simulink model "Simulator_tiltrotor"  (R2016b)
settings: Solver=ode45  StartTime=0.0  StopTime=simulation_time  RelTol=1e-3  EnableMultiTasking=on
InitFcn:
  | Parameters_physical_tiltrotor
undefined symbols (not defined in the file or in its folder): A_Servo, B_Servo, C_Servo, delay_attitude, delay_position, dLMN, gravity, inertia_rotor_hub, inertia_tensor, inertia_tensor_inv, Kq, Kt, mass, mass_matrix, mass_matrix_inv, motor_ome_vs_throttle, motor_tau, sample_time, sigbuilder_block
libraries: aerolibutil x10
(part 1 of 2)
settings Model: Creator=Mattia  LastModifiedBy=Mattia
settings DataIOCC: SaveFormat=Array
settings OptimizationCC: LifeSpan=inf
settings DebuggingCC: SFUnexpectedBacktrackingDiag=warning  SFNoUnconditionalDefaultTransitionDiag=warning  SFExecutionAtInitializationDiag=none
settings GRTTargetCC: TargetLangStandard=C89/C90 (ANSI)  GeneratePreprocessorConditionals=Disable all
settings ConfigComp: CovMetricSettings=dw  CovHtmlReporting=on  CovSaveCumulativeToWorkspaceVar=on  CovSaveSingleToWorkspaceVar=on  CovExternalEMLEnable=off

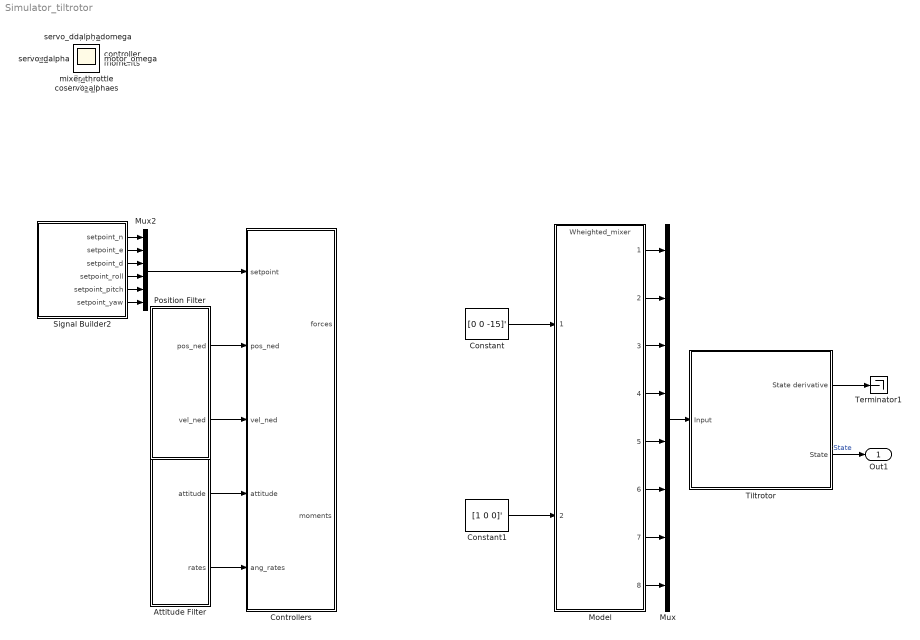
== system Simulator_tiltrotor ==
  Attitude Filter : Subsystem
  Constant : Constant  Value=[0 0 -15]'
  Constant1 : Constant  Value=[1 0 0]'
  Controllers : Subsystem
  Model : ModelReference  ModelNameDialog=Wheighted_mixer.slx  SimulationMode=Normal  ModelReferenceVersion=1.41
  Mux : Mux  Inputs=8
  Mux2 : Mux  Inputs=6
  Position Filter : Subsystem
  Signal Builder2 : Subsystem  Tag=STV Subsys  LoadFcn=sigbuilder_block('load');  StartFcn=sigbuilder_block('start');  StopFcn=sigbuilder_block('stop');  ClipboardFcn=sigbuilder_block('clipboard');  mask(Sigbuilder block){tuvar=[0:10]}
      mask help: Simulink:masks:SigbuilderBlock_MD
      mask init:
      | if ~strcmp(get_param(bdroot(gcbh),'SimulationStatus'),'stopped') tuvar = sigbuilder_block('maskInit'); end
      settings: CopyFcn=sigbuilder_block('copy');  DeleteFcn=sigbuilder_block('delete');  ModelCloseFcn=sigbuilder_block('modelClose');  PreSaveFcn=sigbuilder_block('preSave');  PauseFcn=sigbuilder_block('pause');  ContinueFcn=sigbuilder_block('continue');  NameChangeFcn=sigbuilder_block('namechange');  OpenFcn=sigbuilder_block('open',[6 30 1012.5 447.75 ]);  CloseFcn=sigbuilder_block('close');
      mask Display: plot(0, 0, 100, 100,[2, 2, 32, 32, 2], [68, 8, 8, 68, 68],[32, 2], [38, 38], [32, 19, 2],[53, 60, 44], [32, 17, 17, 2],[16, 16, 31, 31]);txt = getActiveGroup(gcbh);text(2, 100, txt,'verticalAlignment', 'top');
  Terminator1 : Terminator
  Tiltrotor : Subsystem
      mask Display:
      | image(imread('tilt.png'))
      | port_label('input',1,'u')
      | port_label('output',1,'Xdot')
      | port_label('output',2,'X')
  Out1 : Outport
  Fprops : Scope
  Mprops : Scope
  controller_forces : Scope
  controller_moments : Scope
  mixer_alpha : Scope
  mixer_throttle : Scope
  motor_domega : Scope
  motor_omega : Scope
  servo_alpha : Scope
  servo_dalpha : Scope
  servo_ddalpha : Scope
  wires:
  Tiltrotor/1(State derivative) -> Terminator1/1
  Mux/1 -> Tiltrotor/1(Input)
  Tiltrotor/2(State) -> Out1/1  "State"
  Model/1 -> Mux/1
  Model/2 -> Mux/2
  Model/3 -> Mux/3
  Model/4 -> Mux/4
  Model/5 -> Mux/5
  Model/6 -> Mux/6
  Model/7 -> Mux/7
  Model/8 -> Mux/8
  Mux2/1 -> Controllers/1(setpoint)
  Attitude Filter/1(attitude) -> Controllers/4(attitude)
  Attitude Filter/2(rates) -> Controllers/5(ang_rates)
  Position Filter/1(pos_ned) -> Controllers/2(pos_ned)
  Position Filter/2(vel_ned) -> Controllers/3(vel_ned)
  Signal Builder2/3(setpoint_d) -> Mux2/3
  Signal Builder2/4("setpoint_roll ") -> Mux2/4
  Signal Builder2/5(setpoint_pitch) -> Mux2/5
  Signal Builder2/6(setpoint_yaw) -> Mux2/6
  Signal Builder2/2(setpoint_e) -> Mux2/2
  Signal Builder2/1(setpoint_n) -> Mux2/1
  Constant1/1 -> Model/2
  Constant/1 -> Model/1

== system Simulator_tiltrotor/Attitude Filter ==
  Transport Delay : TransportDelay  DelayTime=delay_attitude * sample_time
  Transport Delay1 : TransportDelay  DelayTime=delay_attitude * sample_time
  Zero-Order Hold : ZeroOrderHold  SampleTime=sample_time
  Zero-Order Hold1 : ZeroOrderHold  SampleTime=sample_time
  attitude : Outport  PortDimensions=3
  rates : Outport  Port=2  PortDimensions=3
  wires:
  [ang_rates_body] -> Zero-Order Hold1/1
  [attitude] -> Zero-Order Hold/1
  Zero-Order Hold1/1 -> Transport Delay1/1
  Zero-Order Hold/1 -> Transport Delay/1
  Transport Delay1/1 -> rates/1
  Transport Delay/1 -> attitude/1

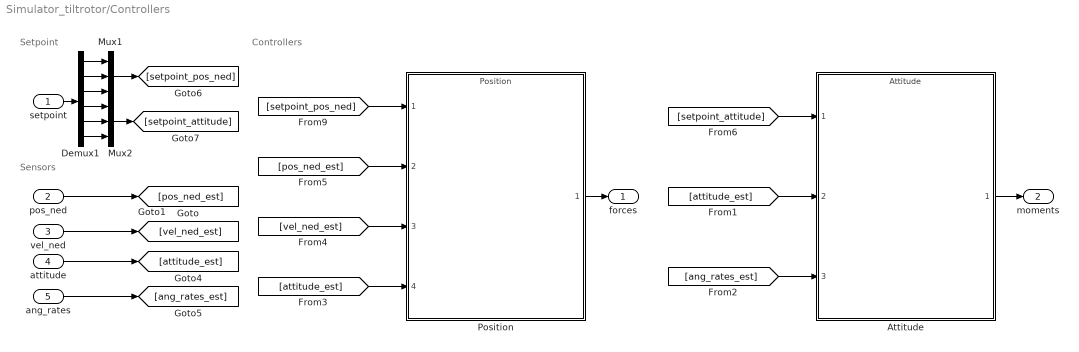
== system Simulator_tiltrotor/Controllers ==
  note: Sensors
  note: Setpoint
  note: Controllers
  setpoint : Inport  PortDimensions=6
  pos_ned : Inport  Port=2  PortDimensions=3
  vel_ned : Inport  Port=3  PortDimensions=3
  attitude : Inport  Port=4  PortDimensions=3
  ang_rates : Inport  Port=5  PortDimensions=3
  Attitude : ModelReference  ModelNameDialog=Attitude.slx  SimulationMode=Normal  ModelReferenceVersion=1.169
  Demux1 : Demux  Outputs=6
  Mux1 : Mux  Inputs=3
  Mux2 : Mux  Inputs=3
  Position : ModelReference  ModelNameDialog=Position.slx  SimulationMode=Normal  ModelReferenceVersion=1.302
  forces : Outport
  moments : Outport  Port=2  PortDimensions=3
  wires:
  setpoint/1 -> Demux1/1
  Demux1/2 -> Mux1/2
  Demux1/1 -> Mux1/1
  [pos_ned_est] -> Position/2
  attitude/1 -> [attitude_est]
  Mux1/1 -> [setpoint_pos_ned]
  [setpoint_pos_ned] -> Position/1
  pos_ned/1 -> [pos_ned_est]
  vel_ned/1 -> [vel_ned_est]
  ang_rates/1 -> [ang_rates_est]
  [attitude_est] -> Position/4
  [vel_ned_est] -> Position/3
  Demux1/3 -> Mux1/3
  Demux1/4 -> Mux2/1
  Demux1/5 -> Mux2/2
  Demux1/6 -> Mux2/3
  Mux2/1 -> [setpoint_attitude]
  Position/1 -> forces/1
  [attitude_est] -> Attitude/2
  Attitude/1 -> moments/1
  [ang_rates_est] -> Attitude/3
  [setpoint_attitude] -> Attitude/1

== system Simulator_tiltrotor/Position Filter ==
  Mux1 : Mux  Inputs=3
  Mux3 : Mux  Inputs=3
  Position NED : Subsystem
  Transport Delay : TransportDelay  DelayTime=delay_position * sample_time
  Transport Delay1 : TransportDelay  DelayTime=delay_position * sample_time
  Velocity NED : Subsystem
  Zero-Order Hold : ZeroOrderHold  SampleTime=sample_time
  Zero-Order Hold1 : ZeroOrderHold  SampleTime=sample_time
  pos_ned : Outport  PortDimensions=3
  vel_ned : Outport  Port=2  PortDimensions=3
  wires:
  Position NED/2(e) -> Mux1/2
  Velocity NED/2(e_vel) -> Mux3/2
  Velocity NED/1(n_vel) -> Mux3/1
  Position NED/1(n) -> Mux1/1
  Zero-Order Hold/1 -> Transport Delay/1
  Mux1/1 -> Zero-Order Hold/1
  Transport Delay/1 -> pos_ned/1
  Zero-Order Hold1/1 -> Transport Delay1/1
  Mux3/1 -> Zero-Order Hold1/1
  Transport Delay1/1 -> vel_ned/1
  Position NED/3(d) -> Mux1/3
  Velocity NED/3(d_vel) -> Mux3/3

== system Simulator_tiltrotor/Signal Builder2 ==
  Demux : Demux  Tag=STV Demux  Outputs=6
  FromWs : FromWorkspace  Tag=STV FromWs  VariableName=tuvar  SampleTime=0
      SigBuilderData=|
      | common.afterFinalStr = 'Extrapolate'
      | common.sampleTime = 0
      | dataSet(1).timeRange = [0 50]
      | dataSet(1).name = 'setpoint'
      | dataSet(2).timeRange = [0 50]
      | dataSet(2).name = 'setpoint_2'
      | sbobj.Groups(1).Name = 'setpoint'
      | sbobj.Groups(1).Signals(1).Name = 'setpoint_n'
      | sbobj.Groups(1).Signals(1).XData = [0 10 13 30 33 50]
      | sbobj.Groups(1).Signals(1).YData = [0 0 1 1 0 0]
      | sbobj.Groups(1).Signals(2).Name = 'setpoint_e'
      | sbobj.Groups(1).Signals(2).XData = [0 50]
      | sbobj.Groups(1).Signals(2).YData = [0 0]
      | sbobj.Groups(1).Signals(3).Name = 'setpoint_d'
      | sbobj.Groups(1).Signals(3).XData = [0 50]
      | sbobj.Groups(1).Signals(3).YData = [-1 -1]
      | sbobj.Groups(1).Signals(4).Name = 'setpoint_roll '
      | sbobj.Groups(1).Signals(4).XData = [0 10 40 50]
      | sbobj.Groups(1).Signals(4).YData = [0 0 0 0]
      | sbobj.Groups(1).Signals(5).Name = 'setpoint_pitch'
      | sbobj.Groups(1).Signals(5).XData = [0 15 16 29 30 50]
      | sbobj.Groups(1).Signals(5).YData = [0 0 1 1 0 0]
      | sbobj.Groups(1).Signals(6).Name = 'setpoint_yaw'
      | sbobj.Groups(1).Signals(6).XData = [0 50]
      | sbobj.Groups(1).Signals(6).YData = [0 0]
      | sbobj.Groups(1).TimeRange = [0 50]
      | sbobj.Groups(2).Name = 'setpoint_2'
      | sbobj.Groups(2).Signals(1).Name = 'setpoint_n'
      | sbobj.Groups(2).Signals(1).XData = [0 10 45 45.05 50]
      | sbobj.Groups(2).Signals(1).YData = [0 0 0 0 0]
      | sbobj.Groups(2).Signals(2).Name = 'setpoint_e'
      | sbobj.Groups(2).Signals(2).XData = [0 10 50]
      | sbobj.Groups(2).Signals(2).YData = [0 0 0]
      | sbobj.Groups(2).Signals(3).Name = 'setpoint_d'
      | sbobj.Groups(2).Signals(3).XData = [0 50]
      | sbobj.Groups(2).Signals(3).YData = [-2 -2]
      | sbobj.Groups(2).Signals(4).Name = 'setpoint_roll '
      | sbobj.Groups(2).Signals(4).XData = [0 10 40 50]
      | sbobj.Groups(2).Signals(4).YData = [0 0 0 0]
      | sbobj.Groups(2).Signals(5).Name = 'setpoint_pitch'
      | sbobj.Groups(2).Signals(5).XData = [0 5 6 14 15 50]
      | sbobj.Groups(2).Signals(5).YData = [0 0 0.314159265359 0.314159265359 0 0]
      | sbobj.Groups(2).Signals(6).Name = 'setpoint_yaw'
      | sbobj.Groups(2).Signals(6).XData = [0 50]
      | sbobj.Groups(2).Signals(6).YData = [0 0]
      | sbobj.Groups(2).TimeRange = [0 50]
  setpoint_n : Outport  Tag=STV Outport
  setpoint_e : Outport  Tag=STV Outport  Port=2
  setpoint_d : Outport  Tag=STV Outport  Port=3
  "setpoint_roll " : Outport  Tag=STV Outport  Port=4
  setpoint_pitch : Outport  Tag=STV Outport  Port=5
  setpoint_yaw : Outport  Tag=STV Outport  Port=6
  wires:
  FromWs/1 -> Demux/1
  Demux/1 -> setpoint_n/1
  Demux/2 -> setpoint_e/1
  Demux/3 -> setpoint_d/1
  Demux/4 -> "setpoint_roll "/1
  Demux/5 -> setpoint_pitch/1
  Demux/6 -> setpoint_yaw/1

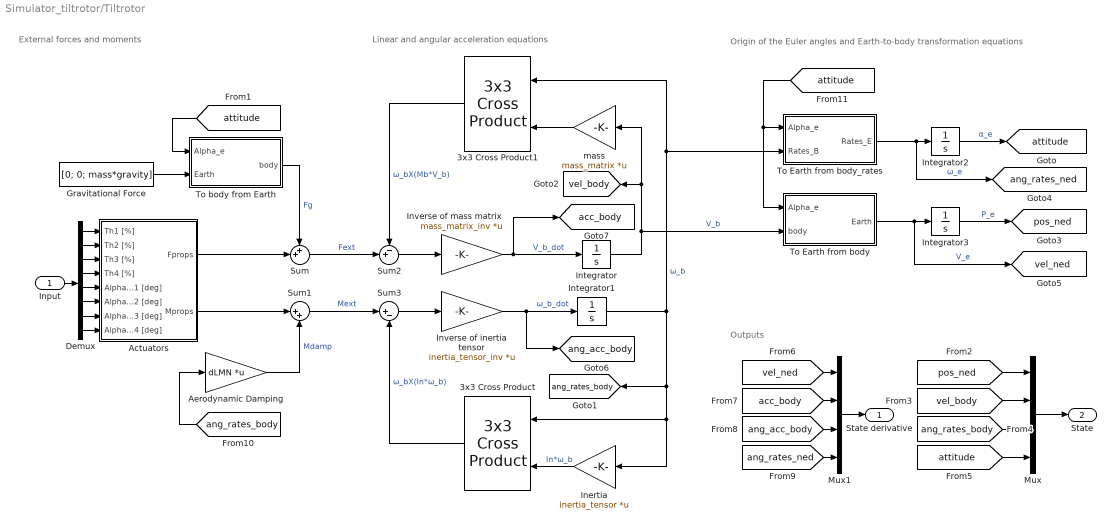
== system Simulator_tiltrotor/Tiltrotor ==
  note: Outputs
  note: Origin of the Euler angles and Earth-to-body transformation equations
  note: Linear and angular acceleration equations
  note: External forces and moments
  Input : Inport
  3x3 Cross Product : aerolibutil/3x3 Cross Product
  3x3 Cross Product1 : aerolibutil/3x3 Cross Product
  Actuators : Subsystem
  Aerodynamic Damping : Gain  Gain=dLMN  Multiplication=Matrix(K*u)
  Demux : Demux  Outputs=8
  Gravitational Force : Constant  Value=[0; 0; mass*gravity]
  Inertia : Gain  Gain=inertia_tensor  Multiplication=Matrix(K*u)
  Integrator{,1..3} (4 alike) : Integrator  InitialCondition=[0; 0; 0]
  Inverse of inertia tensor : Gain  Gain=inertia_tensor_inv  Multiplication=Matrix(K*u)
  Inverse of mass matrix : Gain  Gain=mass_matrix_inv  Multiplication=Matrix(K*u)
  Mux : Mux
  Mux1 : Mux
  Sum : Sum  Inputs=++|
  Sum1 : Sum  Inputs=|++
  Sum2 : Sum  Inputs=-+|
  Sum3 : Sum  Inputs=|+-
  To Earth from body : MATLAB Function  TreatAsAtomicUnit=on
  To Earth from body_rates : MATLAB Function  TreatAsAtomicUnit=on
  To body from Earth : MATLAB Function  TreatAsAtomicUnit=on
  mass : Gain  Gain=mass_matrix  Multiplication=Matrix(K*u)
  State derivative : Outport
  State : Outport  Port=2
  tag scope: acc_body=global, ang_acc_body=global, ang_rates_body=global, ang_rates_ned=global, attitude=global, pos_ned=global, vel_body=global, vel_ned=global
  wires:
  To Earth from body_rates/1(Rates_E) -> Integrator2/1, [ang_rates_ned]  "ω_e"
  [pos_ned] -> Mux/1
  3x3 Cross Product/1 -> Sum3/2  "ω_bX(In*ω_b)"
  [acc_body] -> Mux1/2
  Mux/1 -> State/1
  Mux1/1 -> State derivative/1
  [vel_body] -> Mux/2
  [attitude] -> Mux/4
  [ang_rates_body] -> Mux/3
  [ang_rates_ned] -> Mux1/4
  [ang_acc_body] -> Mux1/3
  [vel_ned] -> Mux1/1
  Inverse of mass matrix/1 -> Integrator/1, [acc_body]  "V_b_dot"
  Integrator/1 -> To Earth from body/2(body), mass/1, [vel_body]  "V_b"
  [attitude] -> To Earth from body/1(Alpha_e), To Earth from body_rates/1(Alpha_e)
  Integrator1/1 -> To Earth from body_rates/2(Rates_B), 3x3 Cross Product1/1, 3x3 Cross Product/1, Inertia/1, [ang_rates_body]  "ω_b"
  Sum3/1 -> Inverse of inertia tensor/1
  Sum2/1 -> Inverse of mass matrix/1
  mass/1 -> 3x3 Cross Product1/2
  Sum/1 -> Sum2/2  "Fext"
  Sum1/1 -> Sum3/1  "Mext"
  Inverse of inertia tensor/1 -> Integrator1/1, [ang_acc_body]  "ω_b_dot"
  3x3 Cross Product1/1 -> Sum2/1  "ω_bX(Mb*V_b)"
  Integrator2/1 -> [attitude]  "α_e"
  Aerodynamic Damping/1 -> Sum1/2  "Mdamp"
  Integrator3/1 -> [pos_ned]  "P_e"
  Inertia/1 -> 3x3 Cross Product/2  "In*ω_b"
  [ang_rates_body] -> Aerodynamic Damping/1
  To Earth from body/1(Earth) -> [vel_ned], Integrator3/1  "V_e"
  To body from Earth/1(body) -> Sum/1  "Fg"
  Gravitational Force/1 -> To body from Earth/2(Earth)
  [attitude] -> To body from Earth/1(Alpha_e)
  Demux/4 -> Actuators/4(Th4 [%])
  Demux/3 -> Actuators/3(Th3 [%])
  Demux/1 -> Actuators/1(Th1 [%])
  Demux/2 -> Actuators/2(Th2 [%])
  Input/1 -> Demux/1
  Demux/5 -> Actuators/5(Alpha_1 [deg])
  Demux/6 -> Actuators/6(Alpha_2 [deg])
  Demux/7 -> Actuators/7(Alpha_3 [deg])
  Demux/8 -> Actuators/8(Alpha_4 [deg])
  Actuators/1(Fprops) -> Sum/2
  Actuators/2(Mprops) -> Sum1/1

== system Simulator_tiltrotor/Position Filter/Position NED ==
  Demux : Demux  Outputs=3
  n : Outport
  e : Outport  Port=2
  d : Outport  Port=3
  wires:
  Demux/1 -> n/1  "n"
  Demux/3 -> d/1  "d"
  [pos_ned] -> Demux/1
  Demux/2 -> e/1  "e"

== system Simulator_tiltrotor/Position Filter/Velocity NED ==
  Demux : Demux  Outputs=3
  n_vel : Outport
  e_vel : Outport  Port=2
  d_vel : Outport  Port=3
  wires:
  Demux/2 -> e_vel/1  "e"
  [vel_ned] -> Demux/1
  Demux/3 -> d_vel/1  "d"
  Demux/1 -> n_vel/1  "n"

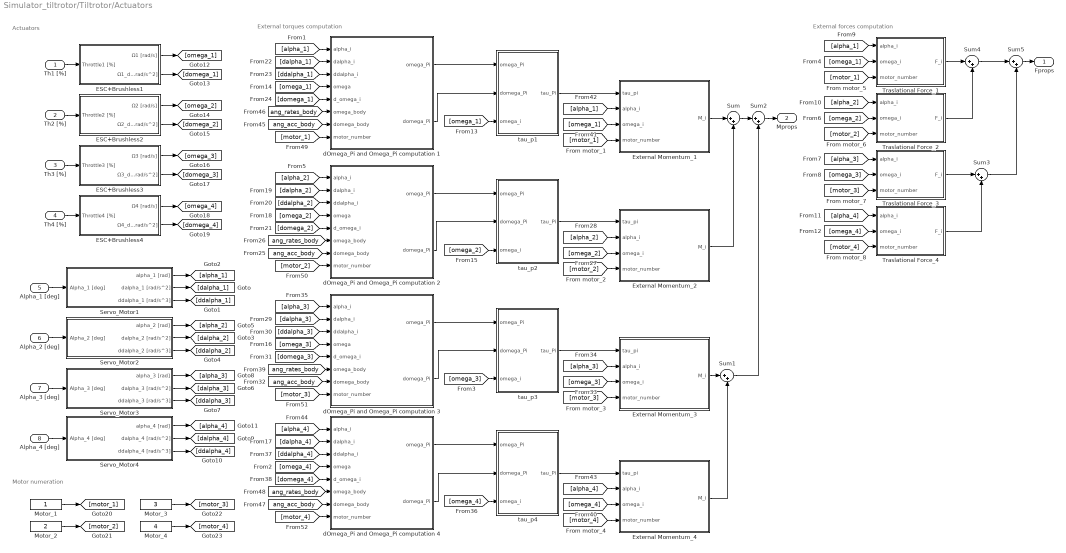
== system Simulator_tiltrotor/Tiltrotor/Actuators ==
  note: Actuators
  note: Motor numeration
  note: External torques computation
  note: External forces computation
  Th1 [%] : Inport
  Th2 [%] : Inport  Port=2
  Th3 [%] : Inport  Port=3
  Th4 [%] : Inport  Port=4
  Alpha_1 [deg] : Inport  Port=5
  Alpha_2 [deg] : Inport  Port=6
  Alpha_3 [deg] : Inport  Port=7
  Alpha_4 [deg] : Inport  Port=8
  ESC+Brushless1 : Subsystem
  ESC+Brushless2 : Subsystem
  ESC+Brushless3 : Subsystem
  ESC+Brushless4 : Subsystem
  External Momentum_1 : Subsystem
  External Momentum_2 : Subsystem
  External Momentum_3 : Subsystem
  External Momentum_4 : Subsystem
  Motor_1 : Constant
  Motor_2 : Constant  Value=2
  Motor_3 : Constant  Value=3
  Motor_4 : Constant  Value=4
  Servo_Motor1 : Subsystem
  Servo_Motor2 : Subsystem
  Servo_Motor3 : Subsystem
  Servo_Motor4 : Subsystem
  Sum{,1..5} (6 alike) : Sum  Inputs=|++
  Traslational Force_1 : Subsystem
  Traslational Force_2 : Subsystem
  Traslational Force_3 : Subsystem
  Traslational Force_4 : Subsystem
  dOmega_Pi and Omega_Pi computation 1 : Subsystem
  dOmega_Pi and Omega_Pi computation 2 : Subsystem
  dOmega_Pi and Omega_Pi computation 3 : Subsystem
  dOmega_Pi and Omega_Pi computation 4 : Subsystem
  tau_p1 : Subsystem
  tau_p2 : Subsystem
  tau_p3 : Subsystem
  tau_p4 : Subsystem
  Fprops : Outport
  Mprops : Outport  Port=2
  wires:
  Th1 [%]/1 -> ESC+Brushless1/1(Throttle1 [%])
  Th2 [%]/1 -> ESC+Brushless2/1(Throttle2 [%])
  Th4 [%]/1 -> ESC+Brushless4/1(Throttle4 [%])
  Th3 [%]/1 -> ESC+Brushless3/1(Throttle3 [%])
  Alpha_1 [deg]/1 -> Servo_Motor1/1(Alpha_1 [deg])
  Servo_Motor1/2(dalpha_1 [rad/s^2]) -> [dalpha_1]
  Servo_Motor1/3(ddalpha_1 [rad/s^3]) -> [ddalpha_1]
  Servo_Motor3/1(alpha_3 [rad]) -> [alpha_3]
  Servo_Motor3/3(ddalpha_3 [rad/s^3]) -> [ddalpha_3]
  Servo_Motor3/2(dalpha_3 [rad/s^2]) -> [dalpha_3]
  Servo_Motor2/3(ddalpha_2 [rad/s^3]) -> [ddalpha_2]
  Servo_Motor2/2(dalpha_2 [rad/s^2]) -> [dalpha_2]
  Servo_Motor2/1(alpha_2 [rad]) -> [alpha_2]
  Servo_Motor1/1(alpha_1 [rad]) -> [alpha_1]
  Servo_Motor4/1(alpha_4 [rad]) -> [alpha_4]
  Servo_Motor4/2(dalpha_4 [rad/s^2]) -> [dalpha_4]
  Servo_Motor4/3(ddalpha_4 [rad/s^3]) -> [ddalpha_4]
  ESC+Brushless1/1(Ω1 [rad/s]) -> [omega_1]
  ESC+Brushless1/2(Ω1_dot [rad/s^2]) -> [domega_1]
  ESC+Brushless2/1(Ω2 [rad/s]) -> [omega_2]
  ESC+Brushless3/1(Ω3 [rad/s]) -> [omega_3]
  ESC+Brushless3/2(Ω3_dot [rad/s^2]) -> [domega_3]
  ESC+Brushless4/1(Ω4 [rad/s]) -> [omega_4]
  ESC+Brushless4/2(Ω4_dot [rad/s^2]) -> [domega_4]
  [alpha_1] -> dOmega_Pi and Omega_Pi computation 1/1(alpha_i)
  [dalpha_1] -> dOmega_Pi and Omega_Pi computation 1/2(dalpha_i)
  [ddalpha_1] -> dOmega_Pi and Omega_Pi computation 1/3(ddalpha_i)
  dOmega_Pi and Omega_Pi computation 1/1(omega_Pi) -> tau_p1/1(omega_Pi)
  dOmega_Pi and Omega_Pi computation 1/2(domega_Pi) -> tau_p1/2(domega_Pi)
  tau_p1/1(tau_Pi) -> External Momentum_1/1(tau_pi)
  [alpha_1] -> External Momentum_1/2(alpha_i)
  [omega_1] -> External Momentum_1/3(omega_i)
  External Momentum_1/1(M_i) -> Sum/1
  Sum/1 -> Sum2/1
  Sum2/1 -> Mprops/1
  [alpha_1] -> Traslational Force_1/1(alpha_i)
  [omega_1] -> Traslational Force_1/2(omega_i)
  Motor_1/1 -> [motor_1]
  Motor_2/1 -> [motor_2]
  Motor_3/1 -> [motor_3]
  Motor_4/1 -> [motor_4]
  Traslational Force_3/1(F_i) -> Sum3/1
  Traslational Force_4/1(F_i) -> Sum3/2
  Traslational Force_1/1(F_i) -> Sum4/1
  Traslational Force_2/1(F_i) -> Sum4/2
  Sum4/1 -> Sum5/1
  Sum3/1 -> Sum5/2
  Sum5/1 -> Fprops/1
  [omega_1] -> tau_p1/3(omega_i)
  Sum1/1 -> Sum2/2
  ESC+Brushless2/2(Ω2_dot [rad/s^2]) -> [domega_2]
  Alpha_2 [deg]/1 -> Servo_Motor2/1(Alpha_2 [deg])
  Alpha_3 [deg]/1 -> Servo_Motor3/1(Alpha_3 [deg])
  Alpha_4 [deg]/1 -> Servo_Motor4/1(Alpha_4 [deg])
  [motor_1] -> External Momentum_1/4(motor_number)
  [alpha_2] -> dOmega_Pi and Omega_Pi computation 2/1(alpha_i)
  [dalpha_2] -> dOmega_Pi and Omega_Pi computation 2/2(dalpha_i)
  [ddalpha_2] -> dOmega_Pi and Omega_Pi computation 2/3(ddalpha_i)
  tau_p2/1(tau_Pi) -> External Momentum_2/1(tau_pi)
  [alpha_2] -> External Momentum_2/2(alpha_i)
  [omega_2] -> External Momentum_2/3(omega_i)
  External Momentum_2/1(M_i) -> Sum/2
  [omega_2] -> tau_p2/3(omega_i)
  [motor_2] -> External Momentum_2/4(motor_number)
  [alpha_3] -> dOmega_Pi and Omega_Pi computation 3/1(alpha_i)
  [dalpha_3] -> dOmega_Pi and Omega_Pi computation 3/2(dalpha_i)
  [ddalpha_3] -> dOmega_Pi and Omega_Pi computation 3/3(ddalpha_i)
  dOmega_Pi and Omega_Pi computation 3/1(omega_Pi) -> tau_p3/1(omega_Pi)
  dOmega_Pi and Omega_Pi computation 3/2(domega_Pi) -> tau_p3/2(domega_Pi)
  [alpha_3] -> External Momentum_3/2(alpha_i)
  [omega_3] -> External Momentum_3/3(omega_i)
  [omega_3] -> tau_p3/3(omega_i)
  [motor_3] -> External Momentum_3/4(motor_number)
  External Momentum_3/1(M_i) -> Sum1/1
  [alpha_4] -> dOmega_Pi and Omega_Pi computation 4/1(alpha_i)
  [dalpha_4] -> dOmega_Pi and Omega_Pi computation 4/2(dalpha_i)
  [ddalpha_4] -> dOmega_Pi and Omega_Pi computation 4/3(ddalpha_i)
  tau_p4/1(tau_Pi) -> External Momentum_4/1(tau_pi)
  [alpha_4] -> External Momentum_4/2(alpha_i)
  [omega_4] -> External Momentum_4/3(omega_i)
  [omega_4] -> tau_p4/3(omega_i)
  [motor_4] -> External Momentum_4/4(motor_number)
  External Momentum_4/1(M_i) -> Sum1/2
  dOmega_Pi and Omega_Pi computation 2/1(omega_Pi) -> tau_p2/1(omega_Pi)
  dOmega_Pi and Omega_Pi computation 2/2(domega_Pi) -> tau_p2/2(domega_Pi)
  [domega_4] -> dOmega_Pi and Omega_Pi computation 4/5(d_omega_i)
  [omega_4] -> dOmega_Pi and Omega_Pi computation 4/4(omega)
  [domega_1] -> dOmega_Pi and Omega_Pi computation 1/5(d_omega_i)
  [omega_1] -> dOmega_Pi and Omega_Pi computation 1/4(omega)
  [ang_rates_body] -> dOmega_Pi and Omega_Pi computation 1/6(omega_body)
  [ang_acc_body] -> dOmega_Pi and Omega_Pi computation 1/7(domega_body)
  [omega_2] -> dOmega_Pi and Omega_Pi computation 2/4(omega)
  [domega_2] -> dOmega_Pi and Omega_Pi computation 2/5(d_omega_i)
  [domega_3] -> dOmega_Pi and Omega_Pi computation 3/5(d_omega_i)
  [omega_3] -> dOmega_Pi and Omega_Pi computation 3/4(omega)
  [ang_rates_body] -> dOmega_Pi and Omega_Pi computation 2/6(omega_body)
  [ang_rates_body] -> dOmega_Pi and Omega_Pi computation 3/6(omega_body)
  [ang_rates_body] -> dOmega_Pi and Omega_Pi computation 4/6(omega_body)
  [ang_acc_body] -> dOmega_Pi and Omega_Pi computation 2/7(domega_body)
  [ang_acc_body] -> dOmega_Pi and Omega_Pi computation 3/7(domega_body)
  [ang_acc_body] -> dOmega_Pi and Omega_Pi computation 4/7(domega_body)
  [motor_1] -> Traslational Force_1/3(motor_number)
  [alpha_2] -> Traslational Force_2/1(alpha_i)
  [alpha_3] -> Traslational Force_3/1(alpha_i)
  [alpha_4] -> Traslational Force_4/1(alpha_i)
  [omega_4] -> Traslational Force_4/2(omega_i)
  [omega_3] -> Traslational Force_3/2(omega_i)
  [motor_2] -> Traslational Force_2/3(motor_number)
  [motor_3] -> Traslational Force_3/3(motor_number)
  [motor_4] -> Traslational Force_4/3(motor_number)
  [omega_2] -> Traslational Force_2/2(omega_i)
  [motor_1] -> dOmega_Pi and Omega_Pi computation 1/8(motor_number)
  dOmega_Pi and Omega_Pi computation 4/1(omega_Pi) -> tau_p4/1(omega_Pi)
  tau_p3/1(tau_Pi) -> External Momentum_3/1(tau_pi)
  dOmega_Pi and Omega_Pi computation 4/2(domega_Pi) -> tau_p4/2(domega_Pi)
  [motor_2] -> dOmega_Pi and Omega_Pi computation 2/8(motor_number)
  [motor_3] -> dOmega_Pi and Omega_Pi computation 3/8(motor_number)
  [motor_4] -> dOmega_Pi and Omega_Pi computation 4/8(motor_number)

== system Simulator_tiltrotor/Tiltrotor/Actuators/ESC+Brushless1 ==
  Throttle1 [%] : Inport
  Gain : Gain
  Gain1 : Gain
  Subsystem : Subsystem
  Ω1 [rad/s] : Outport
  Ω1_dot [rad/s^2] : Outport  Port=2
  wires:
  Subsystem/1(omega_i) -> Gain/1
  Subsystem/2(domega_i) -> Gain1/1
  Throttle1 [%]/1 -> Subsystem/1(Throttle [%])
  Gain/1 -> Ω1 [rad/s]/1
  Gain1/1 -> Ω1_dot [rad/s^2]/1

== system Simulator_tiltrotor/Tiltrotor/Actuators/ESC+Brushless2 ==
  Throttle2 [%] : Inport
  Gain : Gain  Gain=-1
  Gain1 : Gain  Gain=-1
  Subsystem : Subsystem
  Ω2 [rad/s] : Outport
  Ω2_dot [rad/s^2] : Outport  Port=2
  wires:
  Subsystem/1(omega_i) -> Gain/1
  Subsystem/2(domega_i) -> Gain1/1
  Throttle2 [%]/1 -> Subsystem/1(Throttle [%])
  Gain/1 -> Ω2 [rad/s]/1
  Gain1/1 -> Ω2_dot [rad/s^2]/1

== system Simulator_tiltrotor/Tiltrotor/Actuators/ESC+Brushless3 ==
  Throttle3 [%] : Inport
  Gain : Gain
  Gain1 : Gain
  Subsystem : Subsystem
  Ω3 [rad/s] : Outport
  Ω3_dot [rad/s^2] : Outport  Port=2
  wires:
  Subsystem/1(omega_i) -> Gain/1
  Subsystem/2(domega_i) -> Gain1/1
  Throttle3 [%]/1 -> Subsystem/1(Throttle [%])
  Gain/1 -> Ω3 [rad/s]/1
  Gain1/1 -> Ω3_dot [rad/s^2]/1

== system Simulator_tiltrotor/Tiltrotor/Actuators/ESC+Brushless4 ==
  Throttle4 [%] : Inport
  Gain : Gain  Gain=-1
  Gain1 : Gain  Gain=-1
  Subsystem : Subsystem
  Ω4 [rad/s] : Outport
  Ω4_dot [rad/s^2] : Outport  Port=2
  wires:
  Subsystem/1(omega_i) -> Gain/1
  Subsystem/2(domega_i) -> Gain1/1
  Throttle4 [%]/1 -> Subsystem/1(Throttle [%])
  Gain/1 -> Ω4 [rad/s]/1
  Gain1/1 -> Ω4_dot [rad/s^2]/1

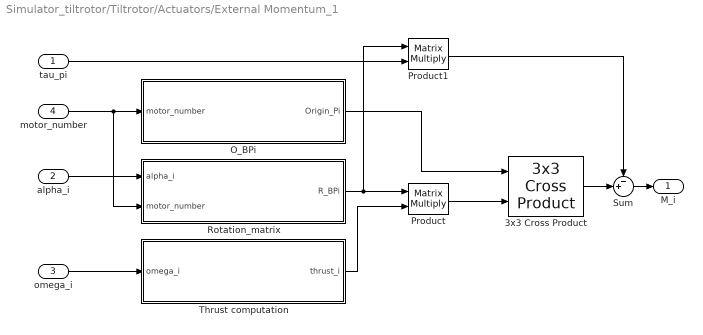
== system Simulator_tiltrotor/Tiltrotor/Actuators/External Momentum_1 ==
  tau_pi : Inport
  alpha_i : Inport  Port=2
  omega_i : Inport  Port=3
  motor_number : Inport  Port=4
  3x3 Cross Product : aerolibutil/3x3 Cross Product
  O_BPi : MATLAB Function  TreatAsAtomicUnit=on
  Product : Product  Multiplication=Matrix(*)
  Product1 : Product  Multiplication=Matrix(*)
  Rotation_matrix : MATLAB Function  TreatAsAtomicUnit=on
  Sum : Sum  Inputs=-+|
  Thrust computation : Subsystem
  M_i : Outport
  wires:
  Sum/1 -> M_i/1
  Rotation_matrix/1(R_BPi) -> Product1/1, Product/1
  alpha_i/1 -> Rotation_matrix/1(alpha_i)
  Product/1 -> 3x3 Cross Product/2
  tau_pi/1 -> Product1/2
  motor_number/1 -> Rotation_matrix/2(motor_number), O_BPi/1(motor_number)
  omega_i/1 -> Thrust computation/1(omega_i)
  Thrust computation/1(thrust_i) -> Product/2
  3x3 Cross Product/1 -> Sum/2
  Product1/1 -> Sum/1
  O_BPi/1(Origin_Pi) -> 3x3 Cross Product/1

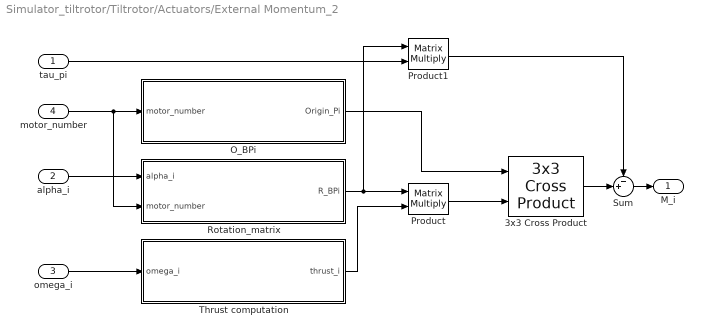
== system Simulator_tiltrotor/Tiltrotor/Actuators/External Momentum_2 ==
  tau_pi : Inport
  alpha_i : Inport  Port=2
  omega_i : Inport  Port=3
  motor_number : Inport  Port=4
  3x3 Cross Product : aerolibutil/3x3 Cross Product
  O_BPi : MATLAB Function  TreatAsAtomicUnit=on
  Product : Product  Multiplication=Matrix(*)
  Product1 : Product  Multiplication=Matrix(*)
  Rotation_matrix : MATLAB Function  TreatAsAtomicUnit=on
  Sum : Sum  Inputs=-+|
  Thrust computation : Subsystem
  M_i : Outport
  wires:
  Sum/1 -> M_i/1
  Rotation_matrix/1(R_BPi) -> Product1/1, Product/1
  alpha_i/1 -> Rotation_matrix/1(alpha_i)
  Product/1 -> 3x3 Cross Product/2
  tau_pi/1 -> Product1/2
  motor_number/1 -> Rotation_matrix/2(motor_number), O_BPi/1(motor_number)
  omega_i/1 -> Thrust computation/1(omega_i)
  Thrust computation/1(thrust_i) -> Product/2
  3x3 Cross Product/1 -> Sum/2
  Product1/1 -> Sum/1
  O_BPi/1(Origin_Pi) -> 3x3 Cross Product/1

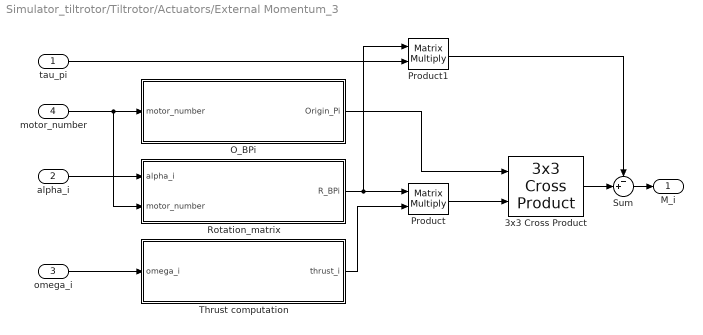
== system Simulator_tiltrotor/Tiltrotor/Actuators/External Momentum_3 ==
  tau_pi : Inport
  alpha_i : Inport  Port=2
  omega_i : Inport  Port=3
  motor_number : Inport  Port=4
  3x3 Cross Product : aerolibutil/3x3 Cross Product
  O_BPi : MATLAB Function  TreatAsAtomicUnit=on
  Product : Product  Multiplication=Matrix(*)
  Product1 : Product  Multiplication=Matrix(*)
  Rotation_matrix : MATLAB Function  TreatAsAtomicUnit=on
  Sum : Sum  Inputs=-+|
  Thrust computation : Subsystem
  M_i : Outport
  wires:
  Sum/1 -> M_i/1
  Rotation_matrix/1(R_BPi) -> Product1/1, Product/1
  alpha_i/1 -> Rotation_matrix/1(alpha_i)
  Product/1 -> 3x3 Cross Product/2
  tau_pi/1 -> Product1/2
  motor_number/1 -> Rotation_matrix/2(motor_number), O_BPi/1(motor_number)
  omega_i/1 -> Thrust computation/1(omega_i)
  Thrust computation/1(thrust_i) -> Product/2
  3x3 Cross Product/1 -> Sum/2
  Product1/1 -> Sum/1
  O_BPi/1(Origin_Pi) -> 3x3 Cross Product/1

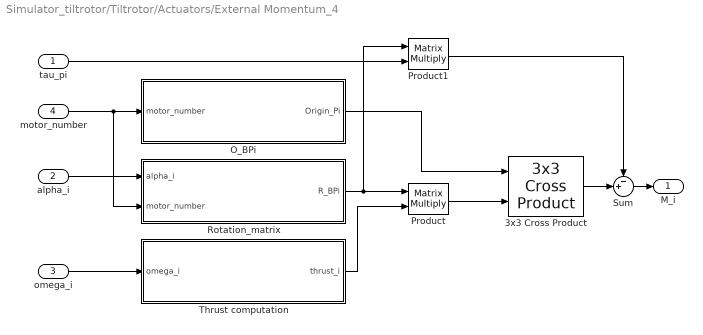
== system Simulator_tiltrotor/Tiltrotor/Actuators/External Momentum_4 ==
  tau_pi : Inport
  alpha_i : Inport  Port=2
  omega_i : Inport  Port=3
  motor_number : Inport  Port=4
  3x3 Cross Product : aerolibutil/3x3 Cross Product
  O_BPi : MATLAB Function  TreatAsAtomicUnit=on
  Product : Product  Multiplication=Matrix(*)
  Product1 : Product  Multiplication=Matrix(*)
  Rotation_matrix : MATLAB Function  TreatAsAtomicUnit=on
  Sum : Sum  Inputs=-+|
  Thrust computation : Subsystem
  M_i : Outport
  wires:
  Sum/1 -> M_i/1
  Rotation_matrix/1(R_BPi) -> Product1/1, Product/1
  alpha_i/1 -> Rotation_matrix/1(alpha_i)
  Product/1 -> 3x3 Cross Product/2
  tau_pi/1 -> Product1/2
  motor_number/1 -> Rotation_matrix/2(motor_number), O_BPi/1(motor_number)
  omega_i/1 -> Thrust computation/1(omega_i)
  Thrust computation/1(thrust_i) -> Product/2
  3x3 Cross Product/1 -> Sum/2
  Product1/1 -> Sum/1
  O_BPi/1(Origin_Pi) -> 3x3 Cross Product/1

== system Simulator_tiltrotor/Tiltrotor/Actuators/Servo_Motor1 ==
  Alpha_1 [deg] : Inport
  Demux : Demux  Outputs=3
  State-Space : StateSpace  A=A_Servo  B=B_Servo  C=C_Servo  D=[0 0 0]'  X0=[0 0 0 ]  ContinuousStateAttributes=['alpha' 'dalpha' 'ddalpha']
  deg2rad : Gain  Gain=deg2rad
  alpha_1 [rad] : Outport
  dalpha_1 [rad/s^2] : Outport  Port=2
  ddalpha_1 [rad/s^3] : Outport  Port=3
  wires:
  deg2rad/1 -> State-Space/1
  Alpha_1 [deg]/1 -> deg2rad/1
  State-Space/1 -> Demux/1
  Demux/1 -> alpha_1 [rad]/1
  Demux/2 -> dalpha_1 [rad/s^2]/1
  Demux/3 -> ddalpha_1 [rad/s^3]/1

== system Simulator_tiltrotor/Tiltrotor/Actuators/Servo_Motor2 ==
  Alpha_2 [deg] : Inport
  Demux : Demux  Outputs=3
  State-Space : StateSpace  A=A_Servo  B=B_Servo  C=C_Servo  D=[0 0 0]'  X0=[0 0 0 ]  ContinuousStateAttributes=['alpha' 'dalpha' 'ddalpha']
  deg2rad : Gain  Gain=deg2rad
  alpha_2 [rad] : Outport
  dalpha_2 [rad/s^2] : Outport  Port=2
  ddalpha_2 [rad/s^3] : Outport  Port=3
  wires:
  deg2rad/1 -> State-Space/1
  Alpha_2 [deg]/1 -> deg2rad/1
  State-Space/1 -> Demux/1
  Demux/1 -> alpha_2 [rad]/1
  Demux/2 -> dalpha_2 [rad/s^2]/1
  Demux/3 -> ddalpha_2 [rad/s^3]/1

== system Simulator_tiltrotor/Tiltrotor/Actuators/Servo_Motor3 ==
  Alpha_3 [deg] : Inport
  Demux : Demux  Outputs=3
  State-Space : StateSpace  A=A_Servo  B=B_Servo  C=C_Servo  D=[0 0 0]'  X0=[0 0 0 ]  ContinuousStateAttributes=['alpha' 'dalpha' 'ddalpha']
  deg2rad : Gain  Gain=deg2rad
  alpha_3 [rad] : Outport
  dalpha_3 [rad/s^2] : Outport  Port=2
  ddalpha_3 [rad/s^3] : Outport  Port=3
  wires:
  deg2rad/1 -> State-Space/1
  Alpha_3 [deg]/1 -> deg2rad/1
  State-Space/1 -> Demux/1
  Demux/1 -> alpha_3 [rad]/1
  Demux/2 -> dalpha_3 [rad/s^2]/1
  Demux/3 -> ddalpha_3 [rad/s^3]/1

== system Simulator_tiltrotor/Tiltrotor/Actuators/Servo_Motor4 ==
  Alpha_4 [deg] : Inport
  Demux : Demux  Outputs=3
  State-Space : StateSpace  A=A_Servo  B=B_Servo  C=C_Servo  D=[0 0 0]'  X0=[0 0 0 ]  ContinuousStateAttributes=['alpha' 'dalpha' 'ddalpha']
  deg2rad : Gain  Gain=deg2rad
  alpha_4 [rad] : Outport
  dalpha_4 [rad/s^2] : Outport  Port=2
  ddalpha_4 [rad/s^3] : Outport  Port=3
  wires:
  deg2rad/1 -> State-Space/1
  Alpha_4 [deg]/1 -> deg2rad/1
  State-Space/1 -> Demux/1
  Demux/1 -> alpha_4 [rad]/1
  Demux/2 -> dalpha_4 [rad/s^2]/1
  Demux/3 -> ddalpha_4 [rad/s^3]/1

== system Simulator_tiltrotor/Tiltrotor/Actuators/Traslational Force_1 ==
  alpha_i : Inport
  omega_i : Inport  Port=2
  motor_number : Inport  Port=3
  Product : Product  Multiplication=Matrix(*)
  Rotation_matrix : MATLAB Function  TreatAsAtomicUnit=on
  Thrust computation : Subsystem
  F_i : Outport
  wires:
  Thrust computation/1(thrust_i) -> Product/2
  Product/1 -> F_i/1
  omega_i/1 -> Thrust computation/1(omega_i)
  Rotation_matrix/1(R_BPi) -> Product/1
  alpha_i/1 -> Rotation_matrix/1(alpha_i)
  motor_number/1 -> Rotation_matrix/2(motor_number)

== system Simulator_tiltrotor/Tiltrotor/Actuators/Traslational Force_2 ==
  alpha_i : Inport
  omega_i : Inport  Port=2
  motor_number : Inport  Port=3
  Product : Product  Multiplication=Matrix(*)
  Rotation_matrix : MATLAB Function  TreatAsAtomicUnit=on
  Thrust computation : Subsystem
  F_i : Outport
  wires:
  motor_number/1 -> Rotation_matrix/2(motor_number)
  alpha_i/1 -> Rotation_matrix/1(alpha_i)
  Rotation_matrix/1(R_BPi) -> Product/1
  omega_i/1 -> Thrust computation/1(omega_i)
  Product/1 -> F_i/1
  Thrust computation/1(thrust_i) -> Product/2

== system Simulator_tiltrotor/Tiltrotor/Actuators/Traslational Force_3 ==
  alpha_i : Inport
  omega_i : Inport  Port=2
  motor_number : Inport  Port=3
  Product : Product  Multiplication=Matrix(*)
  Rotation_matrix : MATLAB Function  TreatAsAtomicUnit=on
  Thrust computation : Subsystem
  F_i : Outport
  wires:
  Thrust computation/1(thrust_i) -> Product/2
  Product/1 -> F_i/1
  omega_i/1 -> Thrust computation/1(omega_i)
  Rotation_matrix/1(R_BPi) -> Product/1
  alpha_i/1 -> Rotation_matrix/1(alpha_i)
  motor_number/1 -> Rotation_matrix/2(motor_number)

== system Simulator_tiltrotor/Tiltrotor/Actuators/Traslational Force_4 ==
  alpha_i : Inport
  omega_i : Inport  Port=2
  motor_number : Inport  Port=3
  Product : Product  Multiplication=Matrix(*)
  Rotation_matrix : MATLAB Function  TreatAsAtomicUnit=on
  Thrust computation : Subsystem
  F_i : Outport
  wires:
  motor_number/1 -> Rotation_matrix/2(motor_number)
  alpha_i/1 -> Rotation_matrix/1(alpha_i)
  Rotation_matrix/1(R_BPi) -> Product/1
  omega_i/1 -> Thrust computation/1(omega_i)
  Product/1 -> F_i/1
  Thrust computation/1(thrust_i) -> Product/2

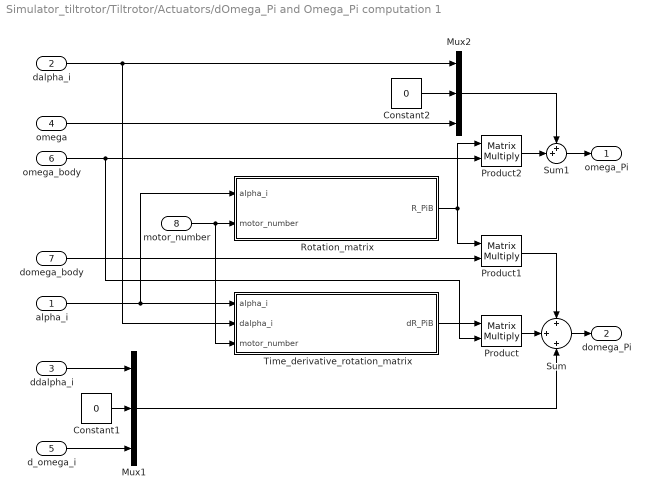
== system Simulator_tiltrotor/Tiltrotor/Actuators/dOmega_Pi and Omega_Pi computation 1 ==
  alpha_i : Inport
  dalpha_i : Inport  Port=2
  ddalpha_i : Inport  Port=3
  omega : Inport  Port=4
  d_omega_i : Inport  Port=5
  omega_body : Inport  Port=6
  domega_body : Inport  Port=7
  motor_number : Inport  Port=8
  Constant1 : Constant  Value=0
  Constant2 : Constant  Value=0
  Mux1 : Mux  Inputs=3
  Mux2 : Mux  Inputs=3
  Product : Product  Multiplication=Matrix(*)
  Product1 : Product  Multiplication=Matrix(*)
  Product2 : Product  Multiplication=Matrix(*)
  Rotation_matrix : MATLAB Function  TreatAsAtomicUnit=on
  Sum : Sum  Inputs=+|+|+
  Sum1 : Sum  Inputs=++|
  Time_derivative_rotation_matrix : MATLAB Function  TreatAsAtomicUnit=on
  omega_Pi : Outport
  domega_Pi : Outport  Port=2
  wires:
  domega_body/1 -> Product1/2
  Product/1 -> Sum/2
  Time_derivative_rotation_matrix/1(dR_PiB) -> Product/1
  Constant1/1 -> Mux1/2
  omega_body/1 -> Product2/2, Product/2
  dalpha_i/1 -> Time_derivative_rotation_matrix/2(dalpha_i), Mux2/1
  alpha_i/1 -> Time_derivative_rotation_matrix/1(alpha_i), Rotation_matrix/1(alpha_i)
  Rotation_matrix/1(R_PiB) -> Product2/1, Product1/1
  Sum/1 -> domega_Pi/1
  Product1/1 -> Sum/1
  Mux1/1 -> Sum/3
  ddalpha_i/1 -> Mux1/1
  Product2/1 -> Sum1/2
  Constant2/1 -> Mux2/2
  Mux2/1 -> Sum1/1
  Sum1/1 -> omega_Pi/1
  d_omega_i/1 -> Mux1/3
  omega/1 -> Mux2/3
  motor_number/1 -> Rotation_matrix/2(motor_number), Time_derivative_rotation_matrix/3(motor_number)

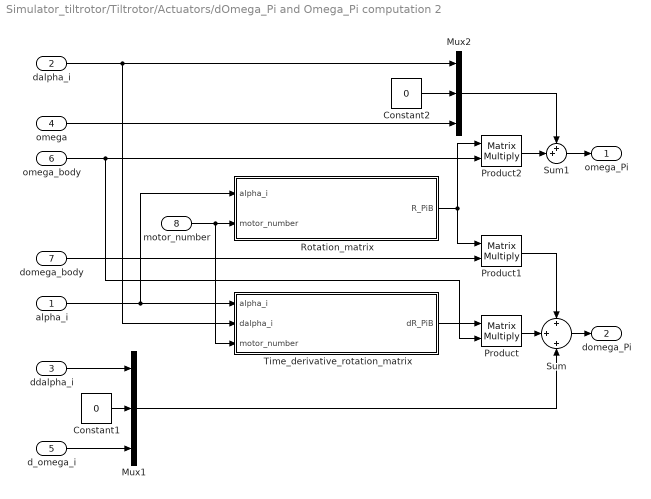
== system Simulator_tiltrotor/Tiltrotor/Actuators/dOmega_Pi and Omega_Pi computation 2 ==
  alpha_i : Inport
  dalpha_i : Inport  Port=2
  ddalpha_i : Inport  Port=3
  omega : Inport  Port=4
  d_omega_i : Inport  Port=5
  omega_body : Inport  Port=6
  domega_body : Inport  Port=7
  motor_number : Inport  Port=8
  Constant1 : Constant  Value=0
  Constant2 : Constant  Value=0
  Mux1 : Mux  Inputs=3
  Mux2 : Mux  Inputs=3
  Product : Product  Multiplication=Matrix(*)
  Product1 : Product  Multiplication=Matrix(*)
  Product2 : Product  Multiplication=Matrix(*)
  Rotation_matrix : MATLAB Function  TreatAsAtomicUnit=on
  Sum : Sum  Inputs=+|+|+
  Sum1 : Sum  Inputs=++|
  Time_derivative_rotation_matrix : MATLAB Function  TreatAsAtomicUnit=on
  omega_Pi : Outport
  domega_Pi : Outport  Port=2
  wires:
  domega_body/1 -> Product1/2
  Product/1 -> Sum/2
  Time_derivative_rotation_matrix/1(dR_PiB) -> Product/1
  Constant1/1 -> Mux1/2
  omega_body/1 -> Product2/2, Product/2
  dalpha_i/1 -> Time_derivative_rotation_matrix/2(dalpha_i), Mux2/1
  alpha_i/1 -> Time_derivative_rotation_matrix/1(alpha_i), Rotation_matrix/1(alpha_i)
  Rotation_matrix/1(R_PiB) -> Product2/1, Product1/1
  Sum/1 -> domega_Pi/1
  Product1/1 -> Sum/1
  Mux1/1 -> Sum/3
  ddalpha_i/1 -> Mux1/1
  Product2/1 -> Sum1/2
  Constant2/1 -> Mux2/2
  Mux2/1 -> Sum1/1
  Sum1/1 -> omega_Pi/1
  d_omega_i/1 -> Mux1/3
  omega/1 -> Mux2/3
  motor_number/1 -> Rotation_matrix/2(motor_number), Time_derivative_rotation_matrix/3(motor_number)

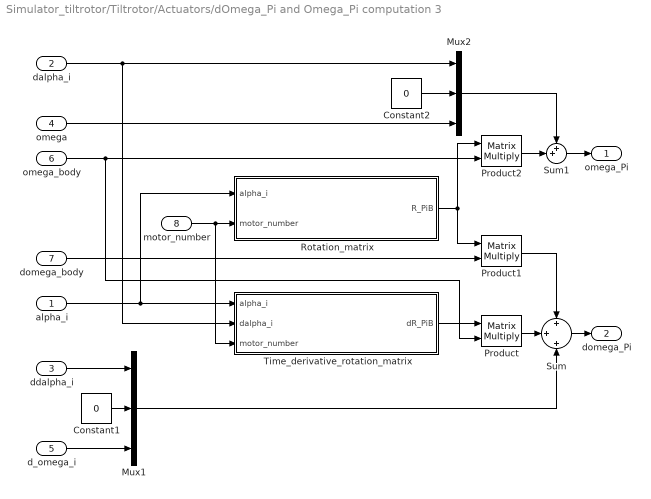
== system Simulator_tiltrotor/Tiltrotor/Actuators/dOmega_Pi and Omega_Pi computation 3 ==
  alpha_i : Inport
  dalpha_i : Inport  Port=2
  ddalpha_i : Inport  Port=3
  omega : Inport  Port=4
  d_omega_i : Inport  Port=5
  omega_body : Inport  Port=6
  domega_body : Inport  Port=7
  motor_number : Inport  Port=8
  Constant1 : Constant  Value=0
  Constant2 : Constant  Value=0
  Mux1 : Mux  Inputs=3
  Mux2 : Mux  Inputs=3
  Product : Product  Multiplication=Matrix(*)
  Product1 : Product  Multiplication=Matrix(*)
  Product2 : Product  Multiplication=Matrix(*)
  Rotation_matrix : MATLAB Function  TreatAsAtomicUnit=on
  Sum : Sum  Inputs=+|+|+
  Sum1 : Sum  Inputs=++|
  Time_derivative_rotation_matrix : MATLAB Function  TreatAsAtomicUnit=on
  omega_Pi : Outport
  domega_Pi : Outport  Port=2
  wires:
  domega_body/1 -> Product1/2
  Product/1 -> Sum/2
  Time_derivative_rotation_matrix/1(dR_PiB) -> Product/1
  Constant1/1 -> Mux1/2
  omega_body/1 -> Product2/2, Product/2
  dalpha_i/1 -> Time_derivative_rotation_matrix/2(dalpha_i), Mux2/1
  alpha_i/1 -> Time_derivative_rotation_matrix/1(alpha_i), Rotation_matrix/1(alpha_i)
  Rotation_matrix/1(R_PiB) -> Product2/1, Product1/1
  Sum/1 -> domega_Pi/1
  Product1/1 -> Sum/1
  Mux1/1 -> Sum/3
  ddalpha_i/1 -> Mux1/1
  Product2/1 -> Sum1/2
  Constant2/1 -> Mux2/2
  Mux2/1 -> Sum1/1
  Sum1/1 -> omega_Pi/1
  d_omega_i/1 -> Mux1/3
  omega/1 -> Mux2/3
  motor_number/1 -> Rotation_matrix/2(motor_number), Time_derivative_rotation_matrix/3(motor_number)

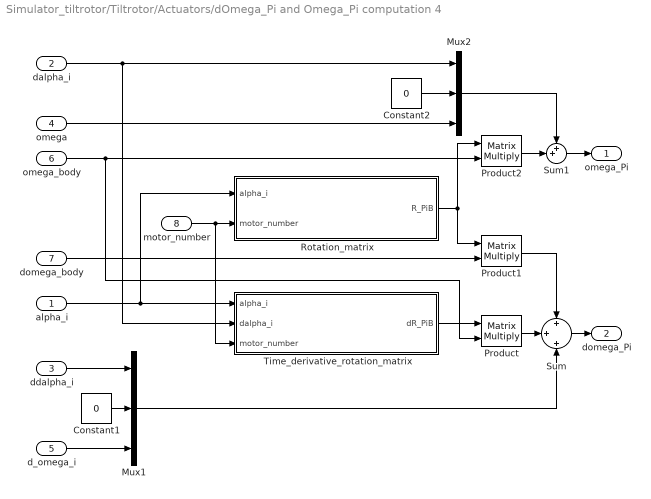
== system Simulator_tiltrotor/Tiltrotor/Actuators/dOmega_Pi and Omega_Pi computation 4 ==
  alpha_i : Inport
  dalpha_i : Inport  Port=2
  ddalpha_i : Inport  Port=3
  omega : Inport  Port=4
  d_omega_i : Inport  Port=5
  omega_body : Inport  Port=6
  domega_body : Inport  Port=7
  motor_number : Inport  Port=8
  Constant1 : Constant  Value=0
  Constant2 : Constant  Value=0
  Mux1 : Mux  Inputs=3
  Mux2 : Mux  Inputs=3
  Product : Product  Multiplication=Matrix(*)
  Product1 : Product  Multiplication=Matrix(*)
  Product2 : Product  Multiplication=Matrix(*)
  Rotation_matrix : MATLAB Function  TreatAsAtomicUnit=on
  Sum : Sum  Inputs=+|+|+
  Sum1 : Sum  Inputs=++|
  Time_derivative_rotation_matrix : MATLAB Function  TreatAsAtomicUnit=on
  omega_Pi : Outport
  domega_Pi : Outport  Port=2
  wires:
  domega_body/1 -> Product1/2
  Product/1 -> Sum/2
  Time_derivative_rotation_matrix/1(dR_PiB) -> Product/1
  Constant1/1 -> Mux1/2
  omega_body/1 -> Product2/2, Product/2
  dalpha_i/1 -> Time_derivative_rotation_matrix/2(dalpha_i), Mux2/1
  alpha_i/1 -> Time_derivative_rotation_matrix/1(alpha_i), Rotation_matrix/1(alpha_i)
  Rotation_matrix/1(R_PiB) -> Product2/1, Product1/1
  Sum/1 -> domega_Pi/1
  Product1/1 -> Sum/1
  Mux1/1 -> Sum/3
  ddalpha_i/1 -> Mux1/1
  Product2/1 -> Sum1/2
  Constant2/1 -> Mux2/2
  Mux2/1 -> Sum1/1
  Sum1/1 -> omega_Pi/1
  d_omega_i/1 -> Mux1/3
  omega/1 -> Mux2/3
  motor_number/1 -> Rotation_matrix/2(motor_number), Time_derivative_rotation_matrix/3(motor_number)

== system Simulator_tiltrotor/Tiltrotor/Actuators/tau_p1 ==
  omega_Pi : Inport
  domega_Pi : Inport  Port=2
  omega_i : Inport  Port=3
  3x3 Cross Product : aerolibutil/3x3 Cross Product
  Constant : Constant  Value=inertia_rotor_hub
  Product : Product  Multiplication=Matrix(*)
  Product1 : Product  Multiplication=Matrix(*)
  Sum : Sum  Inputs=+|+|-
  Torque computation : Subsystem
  tau_Pi : Outport
  wires:
  Constant/1 -> Product/1, Product1/1
  omega_Pi/1 -> Product1/2, 3x3 Cross Product/1
  Product/1 -> Sum/2
  domega_Pi/1 -> Product/2
  Product1/1 -> 3x3 Cross Product/2
  Sum/1 -> tau_Pi/1
  3x3 Cross Product/1 -> Sum/1
  omega_i/1 -> Torque computation/1(omega_i)
  Torque computation/1(torque_i) -> Sum/3

== system Simulator_tiltrotor/Tiltrotor/Actuators/tau_p2 ==
  omega_Pi : Inport
  domega_Pi : Inport  Port=2
  omega_i : Inport  Port=3
  3x3 Cross Product : aerolibutil/3x3 Cross Product
  Constant : Constant  Value=inertia_rotor_hub
  Product : Product  Multiplication=Matrix(*)
  Product1 : Product  Multiplication=Matrix(*)
  Sum : Sum  Inputs=+|+|-
  Torque computation : Subsystem
  tau_Pi : Outport
  wires:
  Constant/1 -> Product/1, Product1/1
  omega_Pi/1 -> Product1/2, 3x3 Cross Product/1
  Product/1 -> Sum/2
  domega_Pi/1 -> Product/2
  Product1/1 -> 3x3 Cross Product/2
  Sum/1 -> tau_Pi/1
  3x3 Cross Product/1 -> Sum/1
  omega_i/1 -> Torque computation/1(omega_i)
  Torque computation/1(torque_i) -> Sum/3

== system Simulator_tiltrotor/Tiltrotor/Actuators/tau_p3 ==
  omega_Pi : Inport
  domega_Pi : Inport  Port=2
  omega_i : Inport  Port=3
  3x3 Cross Product : aerolibutil/3x3 Cross Product
  Constant : Constant  Value=inertia_rotor_hub
  Product : Product  Multiplication=Matrix(*)
  Product1 : Product  Multiplication=Matrix(*)
  Sum : Sum  Inputs=+|+|-
  Torque computation : Subsystem
  tau_Pi : Outport
  wires:
  Constant/1 -> Product/1, Product1/1
  omega_Pi/1 -> Product1/2, 3x3 Cross Product/1
  Product/1 -> Sum/2
  domega_Pi/1 -> Product/2
  Product1/1 -> 3x3 Cross Product/2
  Sum/1 -> tau_Pi/1
  3x3 Cross Product/1 -> Sum/1
  omega_i/1 -> Torque computation/1(omega_i)
  Torque computation/1(torque_i) -> Sum/3

== system Simulator_tiltrotor/Tiltrotor/Actuators/tau_p4 ==
  omega_Pi : Inport
  domega_Pi : Inport  Port=2
  omega_i : Inport  Port=3
  3x3 Cross Product : aerolibutil/3x3 Cross Product
  Constant : Constant  Value=inertia_rotor_hub
  Product : Product  Multiplication=Matrix(*)
  Product1 : Product  Multiplication=Matrix(*)
  Sum : Sum  Inputs=+|+|-
  Torque computation : Subsystem
  tau_Pi : Outport
  wires:
  Constant/1 -> Product/1, Product1/1
  omega_Pi/1 -> Product1/2, 3x3 Cross Product/1
  Product/1 -> Sum/2
  domega_Pi/1 -> Product/2
  Product1/1 -> 3x3 Cross Product/2
  Sum/1 -> tau_Pi/1
  3x3 Cross Product/1 -> Sum/1
  omega_i/1 -> Torque computation/1(omega_i)
  Torque computation/1(torque_i) -> Sum/3

== system Simulator_tiltrotor/Tiltrotor/Actuators/ESC+Brushless1/Subsystem ==
  Throttle [%] : Inport
  Bias : Bias  Bias=motor_ome_vs_throttle(2)
  Gain : Gain  Gain=motor_ome_vs_throttle(1)
  Gain1 : Gain  Gain=-1/motor_tau
  Gain2 : Gain  Gain=1/motor_tau
  Gain3 : Gain  Gain=motor_ome_vs_throttle(1)
  Gain4 : Gain  Gain=motor_ome_vs_throttle(1)
  Sum : Sum  Inputs=|++
  Transfer Fcn : TransferFcn  Denominator=[motor_tau 1]
  Transfer Fcn1 : TransferFcn  Denominator=[motor_tau 1]
  omega_i : Outport
  domega_i : Outport  Port=2
  wires:
  Transfer Fcn1/1 -> Gain1/1
  Gain1/1 -> Gain3/1
  Sum/1 -> domega_i/1
  Gain2/1 -> Gain4/1
  Gain3/1 -> Sum/1
  Bias/1 -> omega_i/1
  Gain/1 -> Bias/1
  Transfer Fcn/1 -> Gain/1
  Throttle [%]/1 -> Gain2/1, Transfer Fcn1/1, Transfer Fcn/1
  Gain4/1 -> Sum/2

== system Simulator_tiltrotor/Tiltrotor/Actuators/ESC+Brushless2/Subsystem ==
  Throttle [%] : Inport
  Bias : Bias  Bias=motor_ome_vs_throttle(2)
  Gain : Gain  Gain=motor_ome_vs_throttle(1)
  Gain1 : Gain  Gain=-1/motor_tau
  Gain2 : Gain  Gain=1/motor_tau
  Gain3 : Gain  Gain=motor_ome_vs_throttle(1)
  Gain4 : Gain  Gain=motor_ome_vs_throttle(1)
  Sum : Sum  Inputs=|++
  Transfer Fcn : TransferFcn  Denominator=[motor_tau 1]
  Transfer Fcn1 : TransferFcn  Denominator=[motor_tau 1]
  omega_i : Outport
  domega_i : Outport  Port=2
  wires:
  Transfer Fcn1/1 -> Gain1/1
  Gain1/1 -> Gain3/1
  Sum/1 -> domega_i/1
  Gain2/1 -> Gain4/1
  Gain3/1 -> Sum/1
  Bias/1 -> omega_i/1
  Gain/1 -> Bias/1
  Transfer Fcn/1 -> Gain/1
  Throttle [%]/1 -> Gain2/1, Transfer Fcn1/1, Transfer Fcn/1
  Gain4/1 -> Sum/2

== system Simulator_tiltrotor/Tiltrotor/Actuators/ESC+Brushless3/Subsystem ==
  Throttle [%] : Inport
  Bias : Bias  Bias=motor_ome_vs_throttle(2)
  Gain : Gain  Gain=motor_ome_vs_throttle(1)
  Gain1 : Gain  Gain=-1/motor_tau
  Gain2 : Gain  Gain=1/motor_tau
  Gain3 : Gain  Gain=motor_ome_vs_throttle(1)
  Gain4 : Gain  Gain=motor_ome_vs_throttle(1)
  Sum : Sum  Inputs=|++
  Transfer Fcn : TransferFcn  Denominator=[motor_tau 1]
  Transfer Fcn1 : TransferFcn  Denominator=[motor_tau 1]
  omega_i : Outport
  domega_i : Outport  Port=2
  wires:
  Transfer Fcn1/1 -> Gain1/1
  Gain1/1 -> Gain3/1
  Sum/1 -> domega_i/1
  Gain2/1 -> Gain4/1
  Gain3/1 -> Sum/1
  Bias/1 -> omega_i/1
  Gain/1 -> Bias/1
  Transfer Fcn/1 -> Gain/1
  Throttle [%]/1 -> Gain2/1, Transfer Fcn1/1, Transfer Fcn/1
  Gain4/1 -> Sum/2

== system Simulator_tiltrotor/Tiltrotor/Actuators/ESC+Brushless4/Subsystem ==
  Throttle [%] : Inport
  Bias : Bias  Bias=motor_ome_vs_throttle(2)
  Gain : Gain  Gain=motor_ome_vs_throttle(1)
  Gain1 : Gain  Gain=-1/motor_tau
  Gain2 : Gain  Gain=1/motor_tau
  Gain3 : Gain  Gain=motor_ome_vs_throttle(1)
  Gain4 : Gain  Gain=motor_ome_vs_throttle(1)
  Sum : Sum  Inputs=|++
  Transfer Fcn : TransferFcn  Denominator=[motor_tau 1]
  Transfer Fcn1 : TransferFcn  Denominator=[motor_tau 1]
  omega_i : Outport
  domega_i : Outport  Port=2
  wires:
  Transfer Fcn1/1 -> Gain1/1
  Gain1/1 -> Gain3/1
  Sum/1 -> domega_i/1
  Gain2/1 -> Gain4/1
  Gain3/1 -> Sum/1
  Bias/1 -> omega_i/1
  Gain/1 -> Bias/1
  Transfer Fcn/1 -> Gain/1
  Throttle [%]/1 -> Gain2/1, Transfer Fcn1/1, Transfer Fcn/1
  Gain4/1 -> Sum/2

== system Simulator_tiltrotor/Tiltrotor/Actuators/External Momentum_1/Thrust computation ==
  omega_i : Inport
  Constant : Constant  Value=-Kt
  Constant1 : Constant  Value=0
  Mux : Mux  Inputs=3
  Product : Product
  Product1 : Product
  thrust_i : Outport
  wires:
  omega_i/1 -> Product/2, Product/1
  Product/1 -> Product1/1
  Constant1/1 -> Mux/2, Mux/1
  Mux/1 -> thrust_i/1
  Product1/1 -> Mux/3
  Constant/1 -> Product1/2

== system Simulator_tiltrotor/Tiltrotor/Actuators/External Momentum_2/Thrust computation ==
  omega_i : Inport
  Constant : Constant  Value=-Kt
  Constant1 : Constant  Value=0
  Mux : Mux  Inputs=3
  Product : Product
  Product1 : Product
  thrust_i : Outport
  wires:
  omega_i/1 -> Product/2, Product/1
  Product/1 -> Product1/1
  Constant1/1 -> Mux/2, Mux/1
  Mux/1 -> thrust_i/1
  Product1/1 -> Mux/3
  Constant/1 -> Product1/2

== system Simulator_tiltrotor/Tiltrotor/Actuators/External Momentum_3/Thrust computation ==
  omega_i : Inport
  Constant : Constant  Value=-Kt
  Constant1 : Constant  Value=0
  Mux : Mux  Inputs=3
  Product : Product
  Product1 : Product
  thrust_i : Outport
  wires:
  omega_i/1 -> Product/2, Product/1
  Product/1 -> Product1/1
  Constant1/1 -> Mux/2, Mux/1
  Mux/1 -> thrust_i/1
  Product1/1 -> Mux/3
  Constant/1 -> Product1/2

== system Simulator_tiltrotor/Tiltrotor/Actuators/External Momentum_4/Thrust computation ==
  omega_i : Inport
  Constant : Constant  Value=-Kt
  Constant1 : Constant  Value=0
  Mux : Mux  Inputs=3
  Product : Product
  Product1 : Product
  thrust_i : Outport
  wires:
  omega_i/1 -> Product/2, Product/1
  Product/1 -> Product1/1
  Constant1/1 -> Mux/2, Mux/1
  Mux/1 -> thrust_i/1
  Product1/1 -> Mux/3
  Constant/1 -> Product1/2

== system Simulator_tiltrotor/Tiltrotor/Actuators/Traslational Force_1/Thrust computation ==
  omega_i : Inport
  Constant : Constant  Value=-Kt
  Constant1 : Constant  Value=0
  Mux : Mux  Inputs=3
  Product : Product
  Product1 : Product
  thrust_i : Outport
  wires:
  omega_i/1 -> Product/2, Product/1
  Product/1 -> Product1/1
  Constant1/1 -> Mux/2, Mux/1
  Mux/1 -> thrust_i/1
  Product1/1 -> Mux/3
  Constant/1 -> Product1/2

== system Simulator_tiltrotor/Tiltrotor/Actuators/Traslational Force_2/Thrust computation ==
  omega_i : Inport
  Constant : Constant  Value=-Kt
  Constant1 : Constant  Value=0
  Mux : Mux  Inputs=3
  Product : Product
  Product1 : Product
  thrust_i : Outport
  wires:
  Constant/1 -> Product1/2
  Product1/1 -> Mux/3
  Mux/1 -> thrust_i/1
  Constant1/1 -> Mux/1, Mux/2
  Product/1 -> Product1/1
  omega_i/1 -> Product/1, Product/2

== system Simulator_tiltrotor/Tiltrotor/Actuators/Traslational Force_3/Thrust computation ==
  omega_i : Inport
  Constant : Constant  Value=-Kt
  Constant1 : Constant  Value=0
  Mux : Mux  Inputs=3
  Product : Product
  Product1 : Product
  thrust_i : Outport
  wires:
  omega_i/1 -> Product/2, Product/1
  Product/1 -> Product1/1
  Constant1/1 -> Mux/2, Mux/1
  Mux/1 -> thrust_i/1
  Product1/1 -> Mux/3
  Constant/1 -> Product1/2

== system Simulator_tiltrotor/Tiltrotor/Actuators/Traslational Force_4/Thrust computation ==
  omega_i : Inport
  Constant : Constant  Value=-Kt
  Constant1 : Constant  Value=0
  Mux : Mux  Inputs=3
  Product : Product
  Product1 : Product
  thrust_i : Outport
  wires:
  Constant/1 -> Product1/2
  Product1/1 -> Mux/3
  Mux/1 -> thrust_i/1
  Constant1/1 -> Mux/1, Mux/2
  Product/1 -> Product1/1
  omega_i/1 -> Product/1, Product/2

== system Simulator_tiltrotor/Tiltrotor/Actuators/tau_p1/Torque computation ==
  omega_i : Inport
  Abs : Abs
  Constant : Constant  Value=-Kq
  Constant1 : Constant  Value=0
  Mux : Mux  Inputs=3
  Product : Product
  Product1 : Product
  torque_i : Outport
  wires:
  omega_i/1 -> Abs/1, Product/2
  Product/1 -> Product1/1
  Constant1/1 -> Mux/2, Mux/1
  Mux/1 -> torque_i/1
  Product1/1 -> Mux/3
  Constant/1 -> Product1/2
  Abs/1 -> Product/1

== system Simulator_tiltrotor/Tiltrotor/Actuators/tau_p2/Torque computation ==
  omega_i : Inport
  Abs : Abs
  Constant : Constant  Value=-Kq
  Constant1 : Constant  Value=0
  Mux : Mux  Inputs=3
  Product : Product
  Product1 : Product
  torque_i : Outport
  wires:
  omega_i/1 -> Abs/1, Product/2
  Product/1 -> Product1/1
  Constant1/1 -> Mux/2, Mux/1
  Mux/1 -> torque_i/1
  Product1/1 -> Mux/3
  Constant/1 -> Product1/2
  Abs/1 -> Product/1

== system Simulator_tiltrotor/Tiltrotor/Actuators/tau_p3/Torque computation ==
  omega_i : Inport
  Abs : Abs
  Constant : Constant  Value=-Kq
  Constant1 : Constant  Value=0
  Mux : Mux  Inputs=3
  Product : Product
  Product1 : Product
  torque_i : Outport
  wires:
  omega_i/1 -> Abs/1, Product/2
  Product/1 -> Product1/1
  Constant1/1 -> Mux/2, Mux/1
  Mux/1 -> torque_i/1
  Product1/1 -> Mux/3
  Constant/1 -> Product1/2
  Abs/1 -> Product/1

== system Simulator_tiltrotor/Tiltrotor/Actuators/tau_p4/Torque computation ==
  omega_i : Inport
  Abs : Abs
  Constant : Constant  Value=-Kq
  Constant1 : Constant  Value=0
  Mux : Mux  Inputs=3
  Product : Product
  Product1 : Product
  torque_i : Outport
  wires:
  omega_i/1 -> Abs/1, Product/2
  Product/1 -> Product1/1
  Constant1/1 -> Mux/2, Mux/1
  Mux/1 -> torque_i/1
  Product1/1 -> Mux/3
  Constant/1 -> Product1/2
  Abs/1 -> Product/1

== matlab function Simulator_tiltrotor/Tiltrotor/To body from Earth ==
  data: Alpha_e input; Earth input; body output
 function body = Tbe(Alpha_e, Earth)
%#codegen
phi = Alpha_e(1);
theta = Alpha_e(2);
psi = Alpha_e(3);

Sphi = sin(phi);
Cphi = cos(phi);
Stheta = sin(theta);
Ctheta = cos(theta);
Spsi = sin(psi);
Cpsi = cos(psi);

TBE = [        Ctheta*Cpsi               Ctheta*Spsi          -Stheta    ;
       Sphi*Stheta*Cpsi-Cphi*Spsi Sphi*Stheta*Spsi+Cphi*Cpsi Sphi*Ctheta ;
       Cphi*Stheta*Cpsi+Sphi*Spsi Cphi*Stheta*Spsi-Sphi*Cpsi Cphi*Ctheta];

body = TBE* Earth;

== matlab function Simulator_tiltrotor/Tiltrotor/To Earth from body ==
  data: Alpha_e input; Earth output; body input
 function Earth = Tbet(Alpha_e, body)
%#codegen
phi = Alpha_e(1);
theta = Alpha_e(2);
psi = Alpha_e(3);

Sphi = sin(phi);
Cphi = cos(phi);
Stheta = sin(theta);
Ctheta = cos(theta);
Spsi = sin(psi);
Cpsi = cos(psi);

TBE = [        Ctheta*Cpsi               Ctheta*Spsi          -Stheta    ;
       Sphi*Stheta*Cpsi-Cphi*Spsi Sphi*Stheta*Spsi+Cphi*Cpsi Sphi*Ctheta ;
       Cphi*Stheta*Cpsi+Sphi*Spsi Cphi*Stheta*Spsi-Sphi*Cpsi Cphi*Ctheta];
TEB = TBE';

Earth = TEB* body;

== matlab function Simulator_tiltrotor/Tiltrotor/To Earth from body_rates ==
  data: Alpha_e input; Rates_B input; Rates_E output
 function Rates_E = Einv(Alpha_e, Rates_B)
%#codegen
phi = Alpha_e(1);
theta = Alpha_e(2);

Sphi = sin(phi);
Cphi = cos(phi);
Ctheta = cos(theta);
Ttheta = tan(theta);

Einv = [1   Sphi*Ttheta    Cphi*Ttheta ;
        0       Cphi          -Sphi    ;
        0   Sphi/Ctheta    Cphi/Ctheta];

Rates_E = Einv* Rates_B;

== matlab function Simulator_tiltrotor/Tiltrotor/Actuators/Traslational Force_1/Rotation_matrix ==
  data: R_BPi output; alpha_i input; motor_number input
function R_BPi = Rotation_matrix( alpha_i, motor_number )
%#codegen
% Rotation matrix from propeller group i-frame to body-frame
phi = alpha_i;
psi = (motor_number - 1) * pi/2;

Sphi = sin(phi);
Cphi = cos(phi);
Spsi = sin(psi);
Cpsi = cos(psi);

Rx = [1   0     0  ;
      0 Cphi -Sphi ;
      0 Sphi  Cphi];
  
Rz = [Cpsi -Spsi 0 ;
      Spsi  Cpsi 0 ;
        0    0   1];
      
R_BPi = Rz * Rx;

== matlab function Simulator_tiltrotor/Tiltrotor/Actuators/External Momentum_2/O_BPi ==
  data: Origin_Pi output; motor_number input; arm_length parameter
 function Origin_Pi = Origin( motor_number, arm_length )
%#codegen
distance = [arm_length ;
                0      ;
                0     ];

psi = (motor_number - 1) * pi/2;

Spsi = sin(psi);
Cpsi = cos(psi);

Rz = [Cpsi -Spsi 0 ;
      Spsi  Cpsi 0 ;
        0    0   1];
      
Origin_Pi = Rz * distance;

== matlab function Simulator_tiltrotor/Tiltrotor/Actuators/External Momentum_2/Rotation_matrix ==
  data: R_BPi output; alpha_i input; motor_number input
function R_BPi = Rotation_matrix( alpha_i, motor_number )
%#codegen
% Rotation matrix from propeller group i-frame to body-frame
phi = alpha_i;
psi = (motor_number - 1) * pi/2;

Sphi = sin(phi);
Cphi = cos(phi);
Spsi = sin(psi);
Cpsi = cos(psi);

Rx = [1   0     0  ;
      0 Cphi -Sphi ;
      0 Sphi  Cphi];
  
Rz = [Cpsi -Spsi 0 ;
      Spsi  Cpsi 0 ;
        0    0   1];
      
R_BPi = Rz * Rx;

== matlab function Simulator_tiltrotor/Tiltrotor/Actuators/dOmega_Pi and Omega_Pi computation 2/Rotation_matrix ==
  data: R_PiB output; alpha_i input; motor_number input
function R_PiB = Rotation_matrix( alpha_i, motor_number )
%#codegen
% Rotation matrix from propeller group i-frame to body-frame
phi = alpha_i;
psi = (motor_number - 1) * pi/2;

Sphi = sin(phi);
Cphi = cos(phi);
Spsi = sin(psi);
Cpsi = cos(psi);

Rx = [1   0     0  ;
      0 Cphi -Sphi ;
      0 Sphi  Cphi];
  
Rz = [Cpsi -Spsi 0 ;
      Spsi  Cpsi 0 ;
        0    0   1];
      
R_BPi = Rz * Rx;
R_PiB = R_BPi';
